simulink model "platoon_model"  (R2018a)
settings: Solver=VariableStepAuto  StartTime=0.0  StopTime=10000.0  RelTol=1e-3
values from neighbouring files (symbols this model uses):
  k_d = 700    [main.m]
  k_i = 0    [main.m]
  k_p = 50    [main.m]
libraries: simulink x1
settings Model: Creator=vxr131730  LastModifiedBy=vxr131730

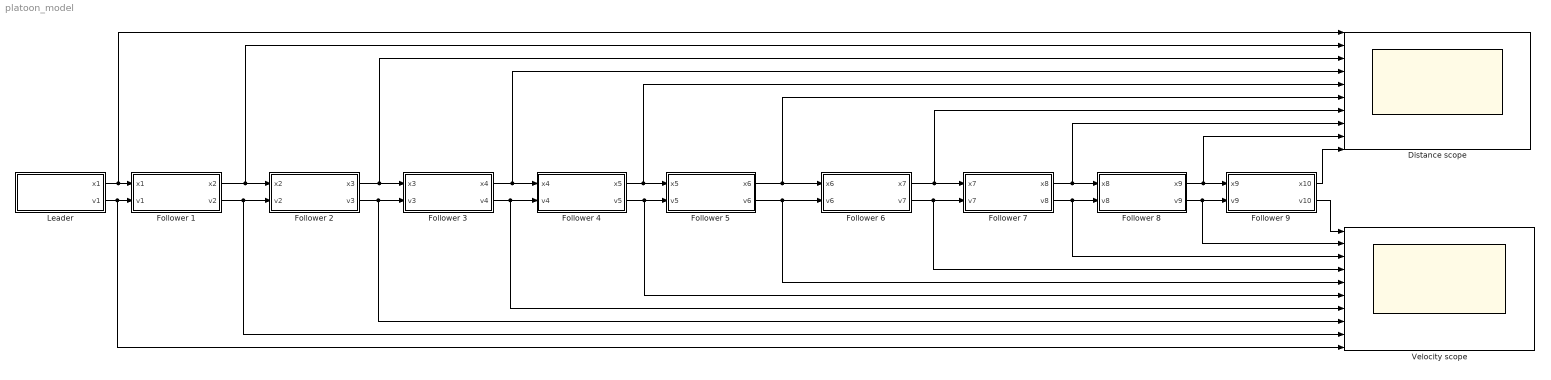
== system platoon_model ==
  Distance scope : Scope  NumInputPorts=10
  Follower 1 : Subsystem
  Follower 2 : Subsystem
  Follower 3 : Subsystem
  Follower 4 : Subsystem
  Follower 5 : Subsystem
  Follower 6 : Subsystem
  Follower 7 : Subsystem
  Follower 8 : Subsystem
  Follower 9 : Subsystem
  Leader : Subsystem
  Velocity scope : Scope  NumInputPorts=10
  wires:
  Leader/1(x1) -> Distance scope/1, Follower 1/1(x1)
  Leader/2(v1) -> Velocity scope/10, Follower 1/2(v1)
  Follower 1/1(x2) -> Distance scope/2, Follower 2/1(x2)
  Follower 1/2(v2) -> Velocity scope/9, Follower 2/2(v2)
  Follower 2/1(x3) -> Distance scope/3, Follower 3/1(x3)
  Follower 2/2(v3) -> Velocity scope/8, Follower 3/2(v3)
  Follower 3/1(x4) -> Distance scope/4, Follower 4/1(x4)
  Follower 3/2(v4) -> Velocity scope/7, Follower 4/2(v4)
  Follower 4/1(x5) -> Distance scope/5, Follower 5/1(x5)
  Follower 4/2(v5) -> Velocity scope/6, Follower 5/2(v5)
  Follower 5/1(x6) -> Distance scope/6, Follower 6/1(x6)
  Follower 5/2(v6) -> Velocity scope/5, Follower 6/2(v6)
  Follower 7/1(x8) -> Distance scope/8, Follower 8/1(x8)
  Follower 7/2(v8) -> Velocity scope/3, Follower 8/2(v8)
  Follower 8/1(x9) -> Distance scope/9, Follower 9/1(x9)
  Follower 8/2(v9) -> Velocity scope/2, Follower 9/2(v9)
  Follower 9/1(x10) -> Distance scope/10
  Follower 9/2(v10) -> Velocity scope/1
  Follower 6/1(x7) -> Distance scope/7, Follower 7/1(x7)
  Follower 6/2(v7) -> Velocity scope/4, Follower 7/2(v7)

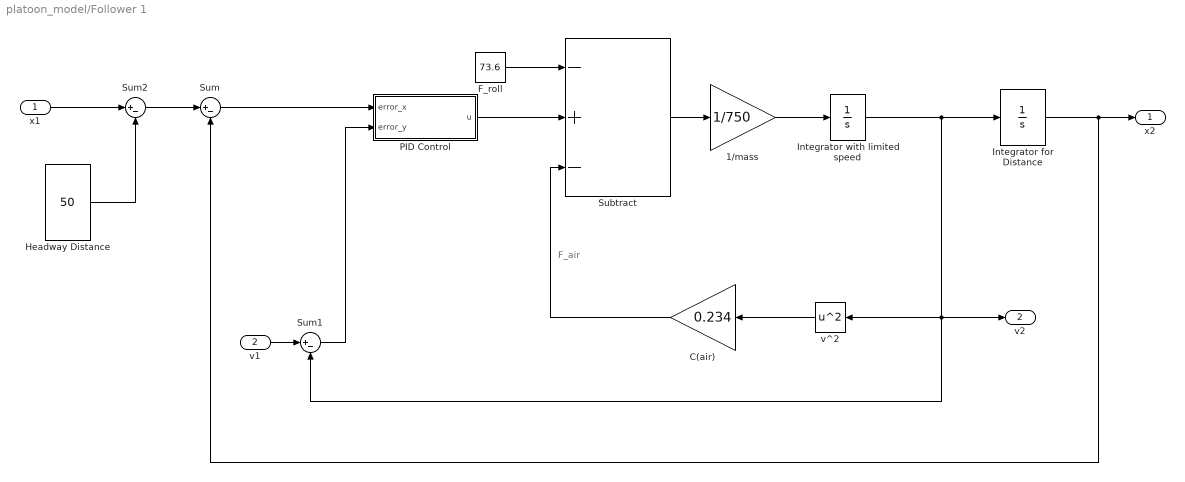
== system platoon_model/Follower 1 ==
  note: F_air
  x1 : Inport
  v1 : Inport  Port=2
  1/mass : Gain  Gain=1/750
  C(air) : Gain  Gain=0.234
  F_roll : Constant  Value=73.6
  Headway Distance : Constant  Value=50
  Integrator with limited speed : Integrator  InitialCondition=20  LimitOutput=on  UpperSaturationLimit=20  LowerSaturationLimit=0
  Integrator for Distance : Integrator  InitialCondition=50
  PID Control : Subsystem
  Subtract : Sum  Inputs=-+-
  Sum : Sum  Inputs=|+-
  Sum1 : Sum  Inputs=|+-
  Sum2 : Sum  Inputs=|+-
  v^2 : Math  Operator=square  SaturateOnIntegerOverflow=on
  x2 : Outport
  v2 : Outport  Port=2
  wires:
  Sum2/1 -> Sum/1
  x1/1 -> Sum2/1
  Subtract/1 -> 1/mass/1
  Integrator with limited speed/1 -> Integrator for Distance/1, v^2/1, v2/1, Sum1/2
  Headway Distance/1 -> Sum2/2
  Integrator for Distance/1 -> x2/1, Sum/2
  F_roll/1 -> Subtract/1
  C(air)/1 -> Subtract/3
  v1/1 -> Sum1/1
  Sum/1 -> PID Control/1(error_x)
  1/mass/1 -> Integrator with limited speed/1
  Sum1/1 -> PID Control/2(error_y)
  v^2/1 -> C(air)/1
  PID Control/1(u) -> Subtract/2

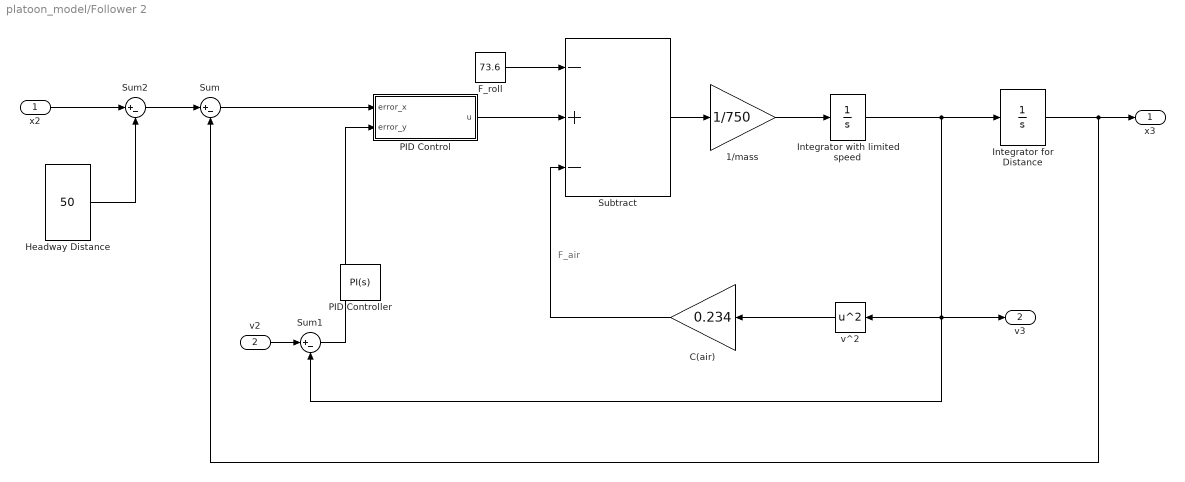
== system platoon_model/Follower 2 ==
  note: F_air
  x2 : Inport
  v2 : Inport  Port=2
  1/mass : Gain  Gain=1/750
  C(air) : Gain  Gain=0.234
  F_roll : Constant  Value=73.6
  Headway Distance : Constant  Value=50
  Integrator with limited speed : Integrator  InitialCondition=20  LimitOutput=on  UpperSaturationLimit=20  LowerSaturationLimit=0
  Integrator for Distance : Integrator  InitialCondition=50
  PID Control : Subsystem
  PID Controller : simulink/Continuous/PID Controller  Controller=PI  TimeDomain=Continuous-time  SampleTime=-1  IntegratorMethod=Forward Euler  FilterMethod=Forward Euler  Form=Parallel  UseFilter=on  ControllerParametersSource=internal  P=1  I=1  D=0  N=100  InitialConditionSource=internal  InitialConditionForIntegrator=0  InitialConditionForFilter=0  ExternalReset=none  LimitOutput=off  UpperSaturationLimit=inf  LowerSaturationLimit=-inf  LinearizeAsGain=on  AntiWindupMode=none  Kb=1  TrackingMode=off  Kt=1  PParamMin=[]  PParamMax=[]  IParamMin=[]  IParamMax=[]  DParamMin=[]  DParamMax=[]  NParamMin=[]  NParamMax=[]  KbParamMin=[]  KbParamMax=[]  KtParamMin=[]  KtParamMax=[]  POutMin=[]  POutMax=[]  IOutMin=[]  IOutMax=[]  DOutMin=[]  DOutMax=[]  NOutMin=[]  NOutMax=[]  KbOutMin=[]  KbOutMax=[]  KtOutMin=[]  KtOutMax=[]  IntegratorOutMin=[]  IntegratorOutMax=[]  FilterOutMin=[]  FilterOutMax=[]  SumOutMin=[]  SumOutMax=[]  SumI1OutMin=[]  SumI1OutMax=[]  SumI2OutMin=[]  SumI2OutMax=[]  SumI3OutMin=[]  SumI3OutMax=[]  SumDOutMin=[]  SumDOutMax=[]  SaturationOutMin=[]  SaturationOutMax=[]  IntegratorContinuousStateAttributes=''  IntegratorStateMustResolveToSignalObject=off  IntegratorRTWStateStorageClass=Auto  FilterContinuousStateAttributes=''  FilterStateMustResolveToSignalObject=off  FilterRTWStateStorageClass=Auto  DifferentiatorICPrevScaledInput=0  DifferentiatorOutMin=[]  DifferentiatorOutMax=[]  FilterDiffOutCoefMin=[]  FilterDiffOutCoefMax=[]  SumDenOutMin=[]  SumDenOutMax=[]  SumNumOutMin=[]  SumNumOutMax=[]  ReciprocalOutMin=[]  ReciprocalOutMax=[]  DivideOutMin=[]  DivideOutMax=[]  TunerSelectOption=Transfer Function Based (PID Tuner App)
  Subtract : Sum  Inputs=-+-
  Sum : Sum  Inputs=|+-
  Sum1 : Sum  Inputs=|+-
  Sum2 : Sum  Inputs=|+-
  v^2 : Math  Operator=square  SaturateOnIntegerOverflow=on
  x3 : Outport
  v3 : Outport  Port=2
  wires:
  PID Control/1(u) -> Subtract/2
  v^2/1 -> C(air)/1
  Sum1/1 -> PID Control/2(error_y)
  1/mass/1 -> Integrator with limited speed/1
  Sum/1 -> PID Control/1(error_x)
  v2/1 -> Sum1/1
  C(air)/1 -> Subtract/3
  F_roll/1 -> Subtract/1
  Integrator for Distance/1 -> Sum/2, x3/1
  Headway Distance/1 -> Sum2/2
  Integrator with limited speed/1 -> v^2/1, Sum1/2, v3/1, Integrator for Distance/1
  Subtract/1 -> 1/mass/1
  x2/1 -> Sum2/1
  Sum2/1 -> Sum/1

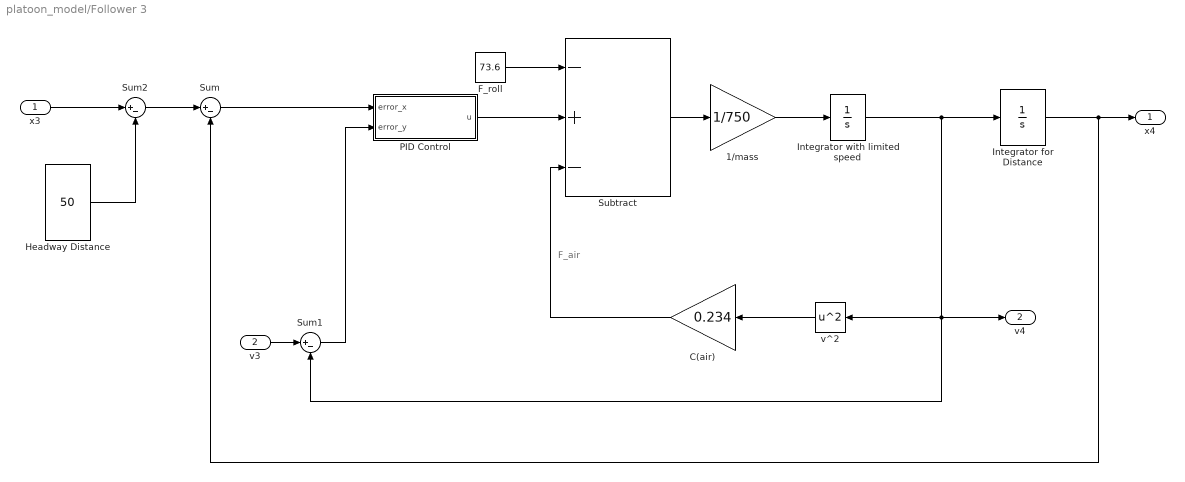
== system platoon_model/Follower 3 ==
  note: F_air
  x3 : Inport
  v3 : Inport  Port=2
  1/mass : Gain  Gain=1/750
  C(air) : Gain  Gain=0.234
  F_roll : Constant  Value=73.6
  Headway Distance : Constant  Value=50
  Integrator with limited speed : Integrator  InitialCondition=20  LimitOutput=on  UpperSaturationLimit=20  LowerSaturationLimit=0
  Integrator for Distance : Integrator  InitialCondition=50
  PID Control : Subsystem
  Subtract : Sum  Inputs=-+-
  Sum : Sum  Inputs=|+-
  Sum1 : Sum  Inputs=|+-
  Sum2 : Sum  Inputs=|+-
  v^2 : Math  Operator=square  SaturateOnIntegerOverflow=on
  x4 : Outport
  v4 : Outport  Port=2
  wires:
  Sum2/1 -> Sum/1
  x3/1 -> Sum2/1
  Subtract/1 -> 1/mass/1
  Integrator with limited speed/1 -> Integrator for Distance/1, v^2/1, v4/1, Sum1/2
  Headway Distance/1 -> Sum2/2
  Integrator for Distance/1 -> x4/1, Sum/2
  F_roll/1 -> Subtract/1
  C(air)/1 -> Subtract/3
  v3/1 -> Sum1/1
  Sum/1 -> PID Control/1(error_x)
  1/mass/1 -> Integrator with limited speed/1
  Sum1/1 -> PID Control/2(error_y)
  v^2/1 -> C(air)/1
  PID Control/1(u) -> Subtract/2

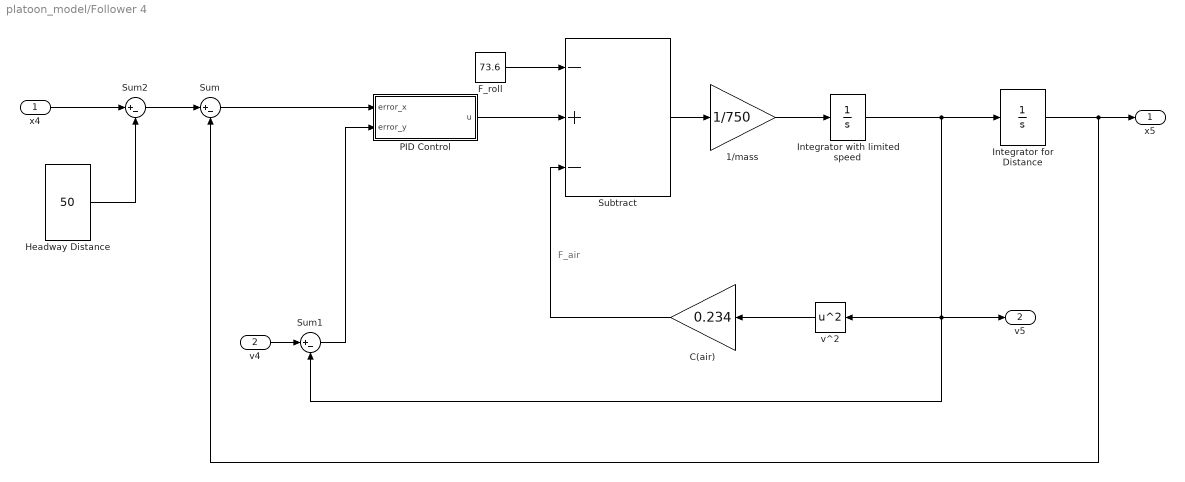
== system platoon_model/Follower 4 ==
  note: F_air
  x4 : Inport
  v4 : Inport  Port=2
  1/mass : Gain  Gain=1/750
  C(air) : Gain  Gain=0.234
  F_roll : Constant  Value=73.6
  Headway Distance : Constant  Value=50
  Integrator with limited speed : Integrator  InitialCondition=20  LimitOutput=on  UpperSaturationLimit=20  LowerSaturationLimit=0
  Integrator for Distance : Integrator  InitialCondition=50
  PID Control : Subsystem
  Subtract : Sum  Inputs=-+-
  Sum : Sum  Inputs=|+-
  Sum1 : Sum  Inputs=|+-
  Sum2 : Sum  Inputs=|+-
  v^2 : Math  Operator=square  SaturateOnIntegerOverflow=on
  x5 : Outport
  v5 : Outport  Port=2
  wires:
  PID Control/1(u) -> Subtract/2
  v^2/1 -> C(air)/1
  Sum1/1 -> PID Control/2(error_y)
  1/mass/1 -> Integrator with limited speed/1
  Sum/1 -> PID Control/1(error_x)
  v4/1 -> Sum1/1
  C(air)/1 -> Subtract/3
  F_roll/1 -> Subtract/1
  Integrator for Distance/1 -> Sum/2, x5/1
  Headway Distance/1 -> Sum2/2
  Integrator with limited speed/1 -> v^2/1, Sum1/2, v5/1, Integrator for Distance/1
  Subtract/1 -> 1/mass/1
  x4/1 -> Sum2/1
  Sum2/1 -> Sum/1

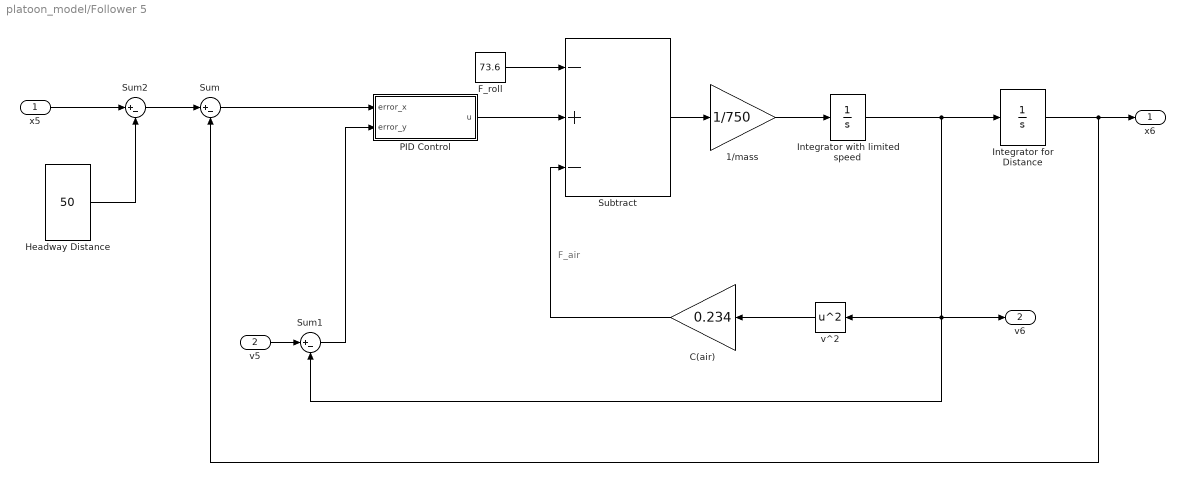
== system platoon_model/Follower 5 ==
  note: F_air
  x5 : Inport
  v5 : Inport  Port=2
  1/mass : Gain  Gain=1/750
  C(air) : Gain  Gain=0.234
  F_roll : Constant  Value=73.6
  Headway Distance : Constant  Value=50
  Integrator with limited speed : Integrator  InitialCondition=20  LimitOutput=on  UpperSaturationLimit=20  LowerSaturationLimit=0
  Integrator for Distance : Integrator  InitialCondition=50
  PID Control : Subsystem
  Subtract : Sum  Inputs=-+-
  Sum : Sum  Inputs=|+-
  Sum1 : Sum  Inputs=|+-
  Sum2 : Sum  Inputs=|+-
  v^2 : Math  Operator=square  SaturateOnIntegerOverflow=on
  x6 : Outport
  v6 : Outport  Port=2
  wires:
  Sum2/1 -> Sum/1
  x5/1 -> Sum2/1
  Subtract/1 -> 1/mass/1
  Integrator with limited speed/1 -> Integrator for Distance/1, v^2/1, v6/1, Sum1/2
  Headway Distance/1 -> Sum2/2
  Integrator for Distance/1 -> x6/1, Sum/2
  F_roll/1 -> Subtract/1
  C(air)/1 -> Subtract/3
  v5/1 -> Sum1/1
  Sum/1 -> PID Control/1(error_x)
  1/mass/1 -> Integrator with limited speed/1
  Sum1/1 -> PID Control/2(error_y)
  v^2/1 -> C(air)/1
  PID Control/1(u) -> Subtract/2

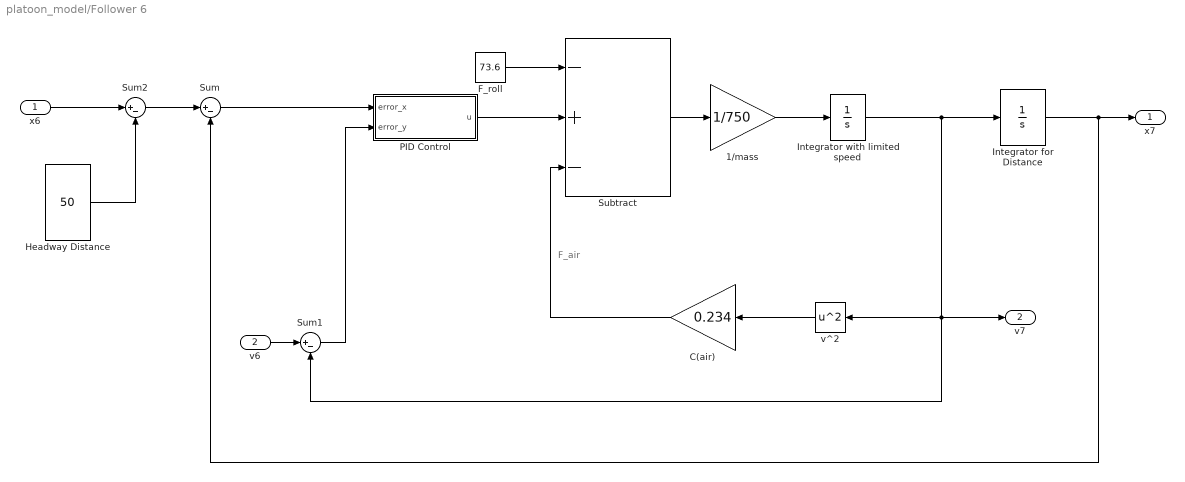
== system platoon_model/Follower 6 ==
  note: F_air
  x6 : Inport
  v6 : Inport  Port=2
  1/mass : Gain  Gain=1/750
  C(air) : Gain  Gain=0.234
  F_roll : Constant  Value=73.6
  Headway Distance : Constant  Value=50
  Integrator with limited speed : Integrator  InitialCondition=20  LimitOutput=on  UpperSaturationLimit=20  LowerSaturationLimit=0
  Integrator for Distance : Integrator  InitialCondition=50
  PID Control : Subsystem
  Subtract : Sum  Inputs=-+-
  Sum : Sum  Inputs=|+-
  Sum1 : Sum  Inputs=|+-
  Sum2 : Sum  Inputs=|+-
  v^2 : Math  Operator=square  SaturateOnIntegerOverflow=on
  x7 : Outport
  v7 : Outport  Port=2
  wires:
  PID Control/1(u) -> Subtract/2
  v^2/1 -> C(air)/1
  Sum1/1 -> PID Control/2(error_y)
  1/mass/1 -> Integrator with limited speed/1
  Sum/1 -> PID Control/1(error_x)
  v6/1 -> Sum1/1
  C(air)/1 -> Subtract/3
  F_roll/1 -> Subtract/1
  Integrator for Distance/1 -> Sum/2, x7/1
  Headway Distance/1 -> Sum2/2
  Integrator with limited speed/1 -> v^2/1, Sum1/2, v7/1, Integrator for Distance/1
  Subtract/1 -> 1/mass/1
  x6/1 -> Sum2/1
  Sum2/1 -> Sum/1

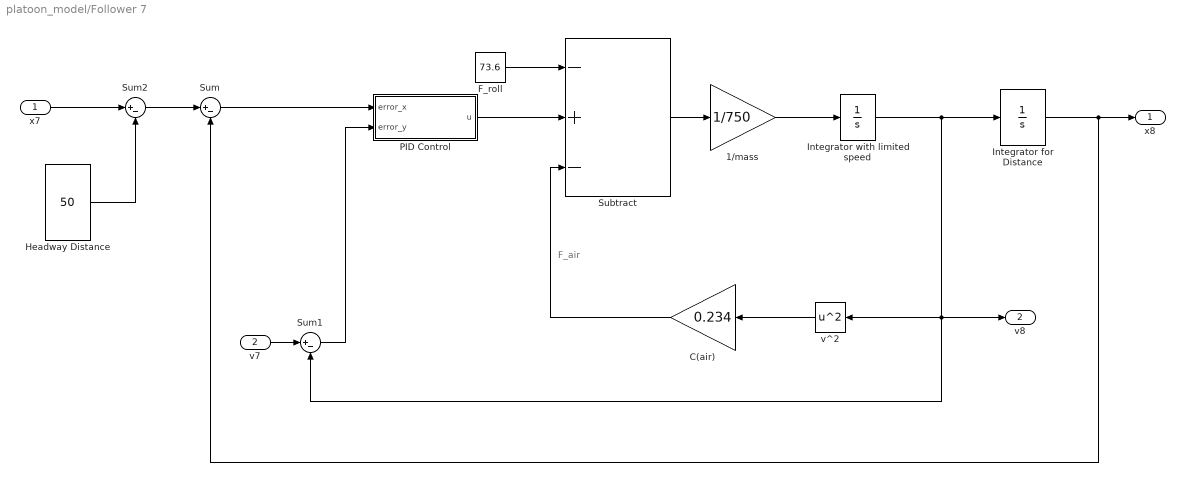
== system platoon_model/Follower 7 ==
  note: F_air
  x7 : Inport
  v7 : Inport  Port=2
  1/mass : Gain  Gain=1/750
  C(air) : Gain  Gain=0.234
  F_roll : Constant  Value=73.6
  Headway Distance : Constant  Value=50
  Integrator with limited speed : Integrator  InitialCondition=20  LimitOutput=on  UpperSaturationLimit=20  LowerSaturationLimit=0
  Integrator for Distance : Integrator  InitialCondition=50
  PID Control : Subsystem
  Subtract : Sum  Inputs=-+-
  Sum : Sum  Inputs=|+-
  Sum1 : Sum  Inputs=|+-
  Sum2 : Sum  Inputs=|+-
  v^2 : Math  Operator=square  SaturateOnIntegerOverflow=on
  x8 : Outport
  v8 : Outport  Port=2
  wires:
  Sum2/1 -> Sum/1
  x7/1 -> Sum2/1
  Subtract/1 -> 1/mass/1
  Integrator with limited speed/1 -> v^2/1, v8/1, Sum1/2, Integrator for Distance/1
  Headway Distance/1 -> Sum2/2
  Integrator for Distance/1 -> x8/1, Sum/2
  F_roll/1 -> Subtract/1
  C(air)/1 -> Subtract/3
  v7/1 -> Sum1/1
  Sum/1 -> PID Control/1(error_x)
  1/mass/1 -> Integrator with limited speed/1
  Sum1/1 -> PID Control/2(error_y)
  v^2/1 -> C(air)/1
  PID Control/1(u) -> Subtract/2

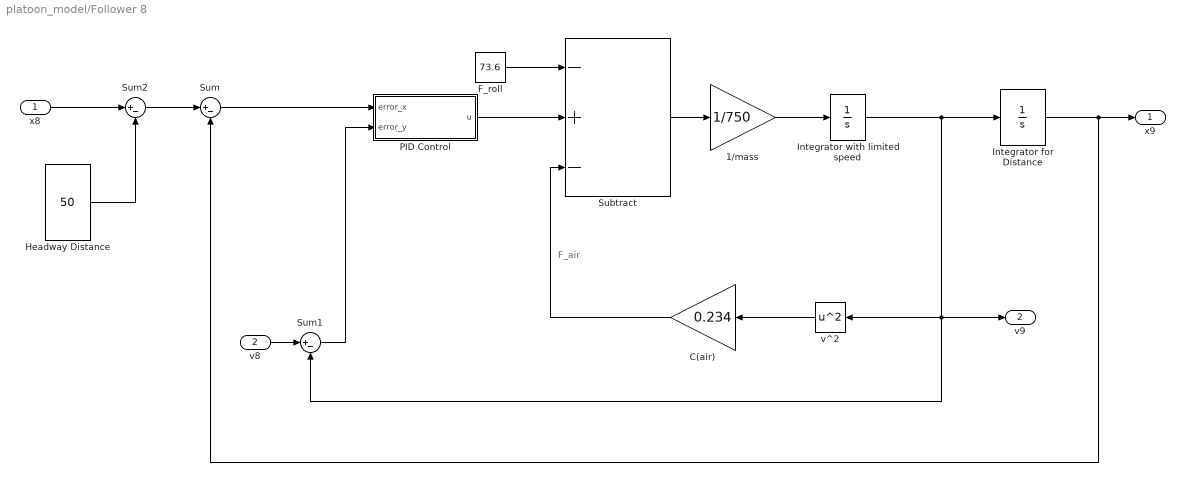
== system platoon_model/Follower 8 ==
  note: F_air
  x8 : Inport
  v8 : Inport  Port=2
  1/mass : Gain  Gain=1/750
  C(air) : Gain  Gain=0.234
  F_roll : Constant  Value=73.6
  Headway Distance : Constant  Value=50
  Integrator with limited speed : Integrator  InitialCondition=20  LimitOutput=on  UpperSaturationLimit=20  LowerSaturationLimit=0
  Integrator for Distance : Integrator  InitialCondition=50
  PID Control : Subsystem
  Subtract : Sum  Inputs=-+-
  Sum : Sum  Inputs=|+-
  Sum1 : Sum  Inputs=|+-
  Sum2 : Sum  Inputs=|+-
  v^2 : Math  Operator=square  SaturateOnIntegerOverflow=on
  x9 : Outport
  v9 : Outport  Port=2
  wires:
  PID Control/1(u) -> Subtract/2
  v^2/1 -> C(air)/1
  Sum1/1 -> PID Control/2(error_y)
  1/mass/1 -> Integrator with limited speed/1
  Sum/1 -> PID Control/1(error_x)
  v8/1 -> Sum1/1
  C(air)/1 -> Subtract/3
  F_roll/1 -> Subtract/1
  Integrator for Distance/1 -> Sum/2, x9/1
  Headway Distance/1 -> Sum2/2
  Integrator with limited speed/1 -> v^2/1, Sum1/2, v9/1, Integrator for Distance/1
  Subtract/1 -> 1/mass/1
  x8/1 -> Sum2/1
  Sum2/1 -> Sum/1

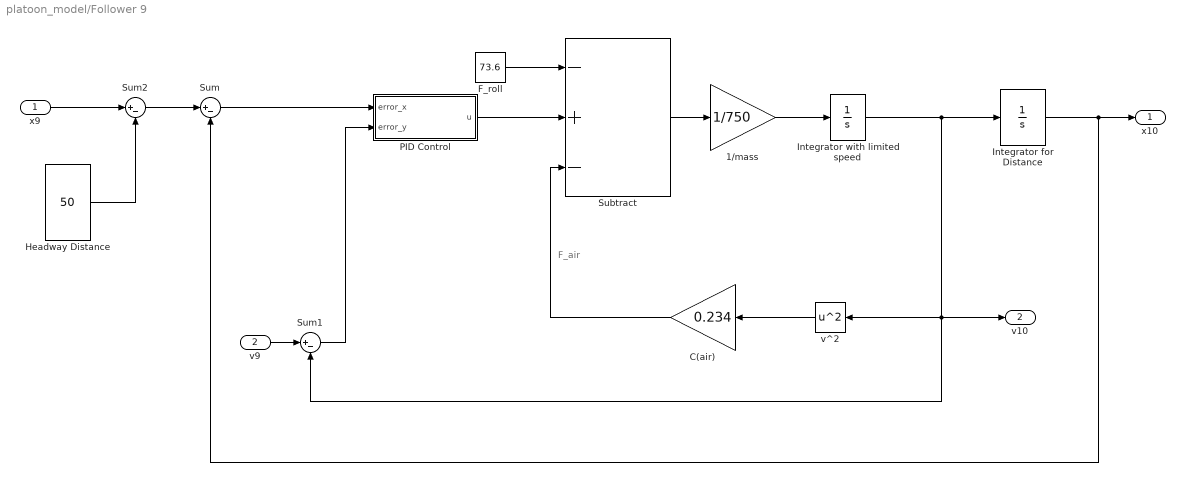
== system platoon_model/Follower 9 ==
  note: F_air
  x9 : Inport
  v9 : Inport  Port=2
  1/mass : Gain  Gain=1/750
  C(air) : Gain  Gain=0.234
  F_roll : Constant  Value=73.6
  Headway Distance : Constant  Value=50
  Integrator with limited speed : Integrator  InitialCondition=20  LimitOutput=on  UpperSaturationLimit=20  LowerSaturationLimit=0
  Integrator for Distance : Integrator  InitialCondition=50
  PID Control : Subsystem
  Subtract : Sum  Inputs=-+-
  Sum : Sum  Inputs=|+-
  Sum1 : Sum  Inputs=|+-
  Sum2 : Sum  Inputs=|+-
  v^2 : Math  Operator=square  SaturateOnIntegerOverflow=on
  x10 : Outport
  v10 : Outport  Port=2
  wires:
  Sum2/1 -> Sum/1
  x9/1 -> Sum2/1
  Subtract/1 -> 1/mass/1
  Integrator with limited speed/1 -> Integrator for Distance/1, v^2/1, v10/1, Sum1/2
  Headway Distance/1 -> Sum2/2
  Integrator for Distance/1 -> x10/1, Sum/2
  F_roll/1 -> Subtract/1
  C(air)/1 -> Subtract/3
  v9/1 -> Sum1/1
  Sum/1 -> PID Control/1(error_x)
  1/mass/1 -> Integrator with limited speed/1
  Sum1/1 -> PID Control/2(error_y)
  v^2/1 -> C(air)/1
  PID Control/1(u) -> Subtract/2

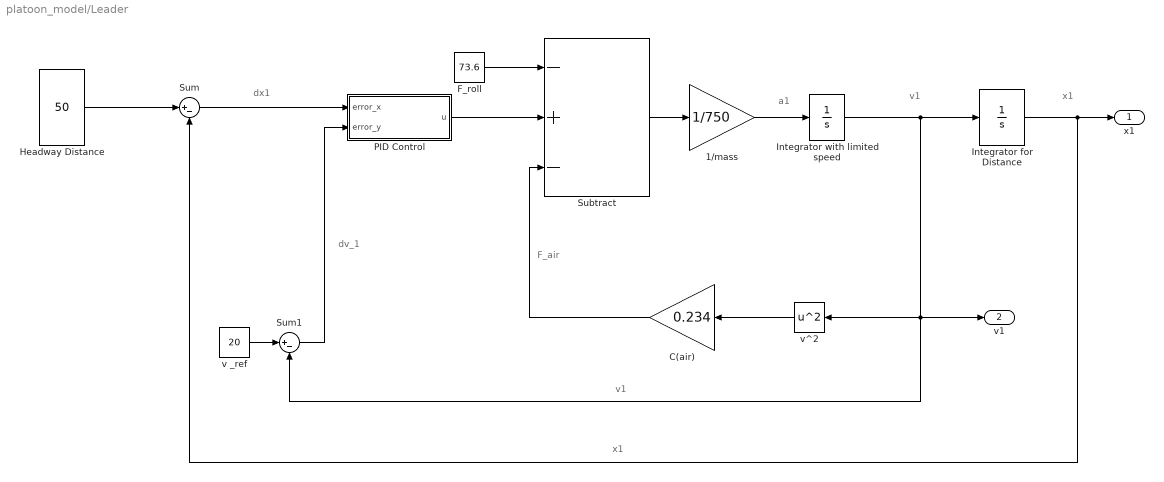
== system platoon_model/Leader ==
  note: a1
  note: dx1
  note: v1
  note: x1
  note: F_air
  note: v1
  note: x1
  note: dv_1
  1/mass : Gain  Gain=1/750
  C(air) : Gain  Gain=0.234
  F_roll : Constant  Value=73.6
  Headway Distance : Constant  Value=50
  Integrator with limited speed : Integrator  InitialCondition=20  LimitOutput=on  UpperSaturationLimit=20  LowerSaturationLimit=0
  Integrator for Distance : Integrator  InitialCondition=50
  PID Control : Subsystem
  Subtract : Sum  Inputs=-+-
  Sum : Sum  Inputs=|+-
  Sum1 : Sum  Inputs=|+-
  v _ref : Constant  Value=20
  v^2 : Math  Operator=square  SaturateOnIntegerOverflow=on
  x1 : Outport
  v1 : Outport  Port=2
  wires:
  v^2/1 -> C(air)/1
  Sum1/1 -> PID Control/2(error_y)
  1/mass/1 -> Integrator with limited speed/1
  Sum/1 -> PID Control/1(error_x)
  C(air)/1 -> Subtract/3
  PID Control/1(u) -> Subtract/2
  F_roll/1 -> Subtract/1
  Integrator for Distance/1 -> Sum/2, x1/1
  Headway Distance/1 -> Sum/1
  Integrator with limited speed/1 -> v^2/1, Sum1/2, v1/1, Integrator for Distance/1
  Subtract/1 -> 1/mass/1
  v _ref/1 -> Sum1/1

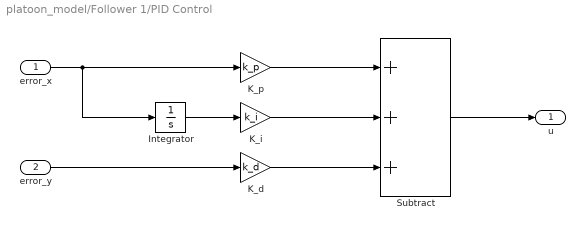
== system platoon_model/Follower 1/PID Control ==
  error_x : Inport
  error_y : Inport  Port=2
  Integrator : Integrator
  K_d : Gain  Gain=k_d
  K_i : Gain  Gain=k_i
  K_p : Gain  Gain=k_p
  Subtract : Sum  Inputs=+++
  u : Outport
  wires:
  Subtract/1 -> u/1
  K_p/1 -> Subtract/1
  K_i/1 -> Subtract/2
  K_d/1 -> Subtract/3
  error_y/1 -> K_d/1
  error_x/1 -> Integrator/1, K_p/1
  Integrator/1 -> K_i/1

== system platoon_model/Follower 2/PID Control ==
  error_x : Inport
  error_y : Inport  Port=2
  Integrator : Integrator
  K_d : Gain  Gain=k_d
  K_i : Gain  Gain=k_i
  K_p : Gain  Gain=k_p
  Subtract : Sum  Inputs=+++
  u : Outport
  wires:
  Integrator/1 -> K_i/1
  error_x/1 -> K_p/1, Integrator/1
  error_y/1 -> K_d/1
  K_d/1 -> Subtract/3
  K_i/1 -> Subtract/2
  K_p/1 -> Subtract/1
  Subtract/1 -> u/1

== system platoon_model/Follower 3/PID Control ==
  error_x : Inport
  error_y : Inport  Port=2
  Integrator : Integrator
  K_d : Gain  Gain=k_d
  K_i : Gain  Gain=k_i
  K_p : Gain  Gain=k_p
  Subtract : Sum  Inputs=+++
  u : Outport
  wires:
  Subtract/1 -> u/1
  K_p/1 -> Subtract/1
  K_i/1 -> Subtract/2
  K_d/1 -> Subtract/3
  error_y/1 -> K_d/1
  error_x/1 -> Integrator/1, K_p/1
  Integrator/1 -> K_i/1

== system platoon_model/Follower 4/PID Control ==
  error_x : Inport
  error_y : Inport  Port=2
  Integrator : Integrator
  K_d : Gain  Gain=k_d
  K_i : Gain  Gain=k_i
  K_p : Gain  Gain=k_p
  Subtract : Sum  Inputs=+++
  u : Outport
  wires:
  Integrator/1 -> K_i/1
  error_x/1 -> K_p/1, Integrator/1
  error_y/1 -> K_d/1
  K_d/1 -> Subtract/3
  K_i/1 -> Subtract/2
  K_p/1 -> Subtract/1
  Subtract/1 -> u/1

== system platoon_model/Follower 5/PID Control ==
  error_x : Inport
  error_y : Inport  Port=2
  Integrator : Integrator
  K_d : Gain  Gain=k_d
  K_i : Gain  Gain=k_i
  K_p : Gain  Gain=k_p
  Subtract : Sum  Inputs=+++
  u : Outport
  wires:
  Subtract/1 -> u/1
  K_p/1 -> Subtract/1
  K_i/1 -> Subtract/2
  K_d/1 -> Subtract/3
  error_y/1 -> K_d/1
  error_x/1 -> Integrator/1, K_p/1
  Integrator/1 -> K_i/1

== system platoon_model/Follower 6/PID Control ==
  error_x : Inport
  error_y : Inport  Port=2
  Integrator : Integrator
  K_d : Gain  Gain=k_d
  K_i : Gain  Gain=k_i
  K_p : Gain  Gain=k_p
  Subtract : Sum  Inputs=+++
  u : Outport
  wires:
  Integrator/1 -> K_i/1
  error_x/1 -> K_p/1, Integrator/1
  error_y/1 -> K_d/1
  K_d/1 -> Subtract/3
  K_i/1 -> Subtract/2
  K_p/1 -> Subtract/1
  Subtract/1 -> u/1

== system platoon_model/Follower 7/PID Control ==
  error_x : Inport
  error_y : Inport  Port=2
  Integrator : Integrator
  K_d : Gain  Gain=k_d
  K_i : Gain  Gain=k_i
  K_p : Gain  Gain=k_p
  Subtract : Sum  Inputs=+++
  u : Outport
  wires:
  Subtract/1 -> u/1
  K_p/1 -> Subtract/1
  K_i/1 -> Subtract/2
  K_d/1 -> Subtract/3
  error_y/1 -> K_d/1
  error_x/1 -> Integrator/1, K_p/1
  Integrator/1 -> K_i/1

== system platoon_model/Follower 8/PID Control ==
  error_x : Inport
  error_y : Inport  Port=2
  Integrator : Integrator
  K_d : Gain  Gain=k_d
  K_i : Gain  Gain=k_i
  K_p : Gain  Gain=k_p
  Subtract : Sum  Inputs=+++
  u : Outport
  wires:
  Integrator/1 -> K_i/1
  error_x/1 -> K_p/1, Integrator/1
  error_y/1 -> K_d/1
  K_d/1 -> Subtract/3
  K_i/1 -> Subtract/2
  K_p/1 -> Subtract/1
  Subtract/1 -> u/1

== system platoon_model/Follower 9/PID Control ==
  error_x : Inport
  error_y : Inport  Port=2
  Integrator : Integrator
  K_d : Gain  Gain=k_d
  K_i : Gain  Gain=k_i
  K_p : Gain  Gain=k_p
  Subtract : Sum  Inputs=+++
  u : Outport
  wires:
  Subtract/1 -> u/1
  K_p/1 -> Subtract/1
  K_i/1 -> Subtract/2
  K_d/1 -> Subtract/3
  error_y/1 -> K_d/1
  error_x/1 -> Integrator/1, K_p/1
  Integrator/1 -> K_i/1

== system platoon_model/Leader/PID Control ==
  error_x : Inport
  error_y : Inport  Port=2
  Integrator : Integrator
  K_d : Gain  Gain=k_d
  K_i : Gain  Gain=k_i
  K_p : Gain  Gain=k_p
  Subtract : Sum  Inputs=+++
  u : Outport
  wires:
  Subtract/1 -> u/1
  K_p/1 -> Subtract/1
  K_i/1 -> Subtract/2
  K_d/1 -> Subtract/3
  error_y/1 -> K_d/1
  error_x/1 -> Integrator/1, K_p/1
  Integrator/1 -> K_i/1
